simulink model "sinlazoalgebraic"  (R2013a)
settings: Solver=ode45  StartTime=0.0  StopTime=100  RelTol=1e-3
values from neighbouring files (symbols this model uses):
  g = 9.81    [miosinlazoalgebraico.m]    (also in yovalores.m)
  theta1 = (m1*lc1*lc1)+(m2*l1*l1)+I1    (= 0.09775488)    [miosinlazoalgebraico.m]
  theta2 = (m2*lc2*lc2)+I2    (= 0.00775807)    [miosinlazoalgebraico.m]
  theta3 = (m2*l1*l2)    (= 0.0287)    [miosinlazoalgebraico.m]
  theta4 = (m1*lc1)+(m2*l1)    (= 0.495148)    [miosinlazoalgebraico.m]
  theta5 = (m2*lc2)    (= 0.044485)    [miosinlazoalgebraico.m]
settings Model: Creator=Daniel  LastModifiedBy=Daniel

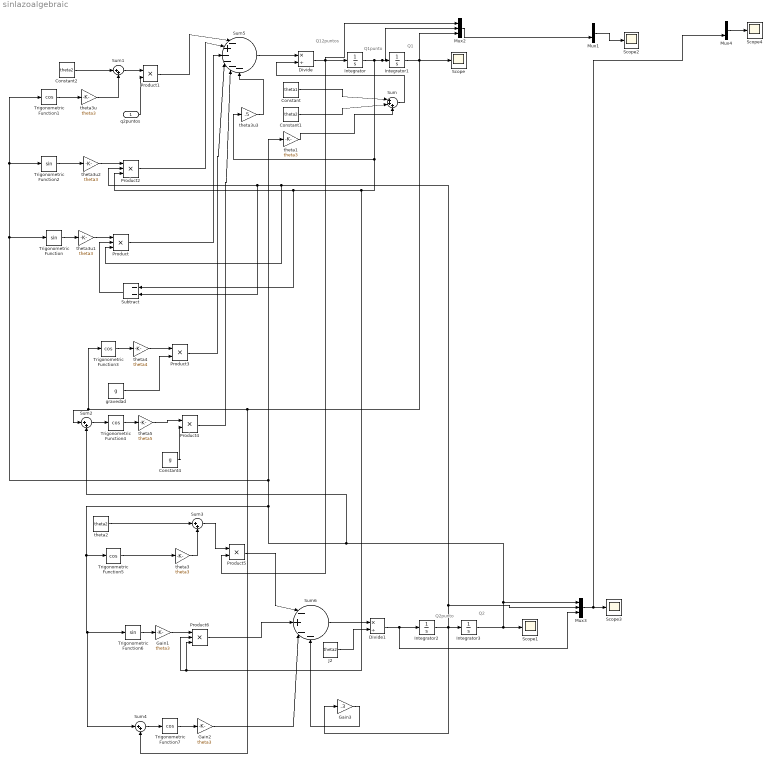
== system sinlazoalgebraic ==
  note: Q1
  note: Q1punto
  note: Q12puntos
  note: Q2
  note: Q2punto
  q2puntos : Inport
  Constant : Constant  Value=theta1
  Constant1 : Constant  Value=theta2
  Constant2 : Constant  Value=theta2
  Constant4 : Constant  Value=g
  Divide : Product  Inputs=*/
  Divide1 : Product  Inputs=*/
  Gain1 : Gain  Gain=theta3
  Gain2 : Gain  Gain=theta3
  Gain3 : Gain  Gain=.3
  Integrator : Integrator
  Integrator1 : Integrator  InitialCondition=pi
  Integrator2 : Integrator
  Integrator3 : Integrator  InitialCondition=pi
  J2 : Constant  Value=theta2
  Mux1 : Mux  Inputs=2
  Mux2 : Mux  Inputs=3
  Mux3 : Mux  Inputs=3
  Mux4 : Mux  Inputs=2
  Product : Product  Inputs=3
  Product{1,3..5} (4 alike) : Product
  Product2 : Product  Inputs=3
  Product6 : Product  Inputs=3
  Scope{,1..4} (5 alike) : Scope
      Scope settings: YMin=4.6966  YMax=4.6981
      Scope1 settings: YMin=2.73642  YMax=2.7365
      Scope2 settings: YMin=4.6966  YMax=4.6981  SaveName=ScopeData2
      Scope3 settings: YMin=2.73642  YMax=2.7365  SaveName=ScopeData3
      Scope4 settings: YMin=4.6966  YMax=4.6981  SaveName=ScopeData4
  Subtract : Sum  Inputs=--
  Sum : Sum  Inputs=|+++
  Sum{1..4} (4 alike) : Sum  Inputs=|++
  Sum5 : Sum  Inputs=|-+----
  Sum6 : Sum  Inputs=|-+--
  Trigonometric Function : Trigonometry
  Trigonometric Function{1,3..5,7} (5 alike) : Trigonometry  Operator=cos
  Trigonometric Function2 : Trigonometry
  Trigonometric Function6 : Trigonometry
  gravedad : Constant  Value=g
  theta1 : Gain  Gain=theta3
  theta2 : Constant  Value=theta2
  theta3 : Gain  Gain=theta3
  theta3u : Gain  Gain=theta3
  theta3u1 : Gain  Gain=theta3
  theta3u2 : Gain  Gain=theta3
  theta3u3 : Gain  Gain=.5
  theta4 : Gain  Gain=theta4
  theta5 : Gain  Gain=theta5
  wires:
  Constant2/1 -> Sum1/1
  theta3u/1 -> Sum1/2
  Trigonometric Function1/1 -> theta3u/1
  Sum1/1 -> Product1/1
  q2puntos/1 -> Product1/2
  Product1/1 -> Sum5/1
  Trigonometric Function2/1 -> theta3u2/1
  theta3u2/1 -> Product2/1
  Product2/1 -> Sum5/2
  Product/1 -> Sum5/3
  Trigonometric Function/1 -> theta3u1/1
  theta3u1/1 -> Product/1
  Product3/1 -> Sum5/4
  Trigonometric Function3/1 -> theta4/1
  theta4/1 -> Product3/1
  gravedad/1 -> Product3/2
  Product4/1 -> Sum5/5
  Trigonometric Function4/1 -> theta5/1
  Sum2/1 -> Trigonometric Function4/1
  theta5/1 -> Product4/1
  Constant4/1 -> Product4/2
  Trigonometric Function5/1 -> theta3/1
  theta2/1 -> Sum3/1
  theta3/1 -> Sum3/2
  Sum3/1 -> Product5/1
  Divide/1 -> Mux2/1, Product5/2, Integrator/1
  Product5/1 -> Sum6/1
  Trigonometric Function6/1 -> Gain1/1
  Product6/1 -> Sum6/2
  Integrator/1 -> Mux2/2, Integrator1/1, theta3u3/1, Product6/3, Product6/2, Subtract/1, Product2/3
  Gain1/1 -> Product6/1
  Gain2/1 -> Sum6/3
  Integrator3/1 -> Mux3/1, Sum2/2, theta1/1, Trigonometric Function/1, Trigonometric Function2/1, Trigonometric Function1/1, Sum4/1, Trigonometric Function6/1, Trigonometric Function5/1, Scope1/1
  Trigonometric Function7/1 -> Gain2/1
  Sum4/1 -> Trigonometric Function7/1
  Integrator1/1 -> Mux2/3, Sum4/2, Trigonometric Function3/1, Sum2/1, Scope/1
  Constant/1 -> Sum/1
  Constant1/1 -> Sum/2
  theta1/1 -> Sum/3
  Sum/1 -> Divide/2
  Sum5/1 -> Divide/1
  Sum6/1 -> Divide1/1
  Divide1/1 -> Mux3/3, Integrator2/1
  J2/1 -> Divide1/2
  Subtract/1 -> Product/2
  theta3u3/1 -> Sum5/6
  Gain3/1 -> Sum6/4
  Mux2/1 -> Mux1/2
  Mux1/1 -> Scope2/1
  Integrator2/1 -> Gain3/1, Mux3/2, Product/3, Subtract/2, Product2/2, Integrator3/1
  Mux3/1 -> Mux4/2, Scope3/1
  Mux4/1 -> Scope4/1
